simulink model "quadcopter_controly_system"  (R2016b)
settings: Solver=FixedStepAuto  StartTime=0.0  StopTime=30  FixedStep=0.001  MaxStep=0.004  RelTol=1e-3
PreLoadFcn:
  | init
model workspace (MAT data in the model file):
  SL_ROS_VariableLengthArrays_MaxSizes.CommonInfo.ArrayTruncateAction = 'EmitWarning'
  SL_ROS_VariableLengthArrays_MaxSizes.MsgTypeMap = containers.Map
  SL_ROS_VariableLengthArrays_MaxSizes.MsgTypeMap.serialization.keys = {}
  SL_ROS_VariableLengthArrays_MaxSizes.MsgTypeMap.serialization.values = {}
  SL_ROS_VariableLengthArrays_MaxSizes.MsgTypeMap.serialization.uniformity = 0
  SL_ROS_VariableLengthArrays_MaxSizes.MsgTypeMap.serialization.keyType = 'char'
  SL_ROS_VariableLengthArrays_MaxSizes.MsgTypeMap.serialization.valueType = 'any'
undefined symbols (not defined in the file or in its folder): Data, Data_SL_Info
libraries: robotlib x3
settings Model: Creator=ADAM  LastModifiedBy=consti
settings SolverCC: ExtrapolationOrder=1
settings DataIOCC: MaxDataPoints=1  SaveFormat=Structure  SignalLoggingSaveFormat=ModelDataLogs  SaveOutput=off  SignalLogging=off  DSMLogging=off  SaveTime=off  OutputSaveName=model_out  SignalLoggingName=model_out
settings OptimizationCC: ExpressionDepthLimit=2147483647  LifeSpan=inf  SimCompilerOptimization=on
settings DebuggingCC: UnderspecifiedInitializationDetection=Classic  MergeDetectMultiDrivingBlocksExec=none  InheritedTsInSrcMsg=none  MultiTaskDSMMsg=warning  MultiTaskCondExecSysMsg=none  UnconnectedInputMsg=none  UnconnectedOutputMsg=none  UnconnectedLineMsg=none  StateNameClashWarn=warning  SFUnexpectedBacktrackingDiag=warning  SFNoUnconditionalDefaultTransitionDiag=warning  SFExecutionAtInitializationDiag=none
settings HardwareCC: ProdBitPerPointer=32  ProdBitPerSizeT=32  ProdBitPerPtrDiffT=32  ProdLargestAtomicFloat=None  ProdWordSize=32  ProdHWDeviceType=Generic->32-bit x86 compatible
settings ModelReferenceCC: UpdateModelReferenceTargets=IfOutOfDate  PropagateSignalLabelsOutOfModel=off
settings CodeAppCC: MaxIdLength=95
settings GRTTargetCC: TargetLangStandard=C89/C90 (ANSI)  GeneratePreprocessorConditionals=Disable all
settings ConfigComp: CovMetricSettings=dw  CovHtmlReporting=on  CovSaveCumulativeToWorkspaceVar=on  CovSaveSingleToWorkspaceVar=on  CovExternalEMLEnable=off  CovSFcnEnable=off

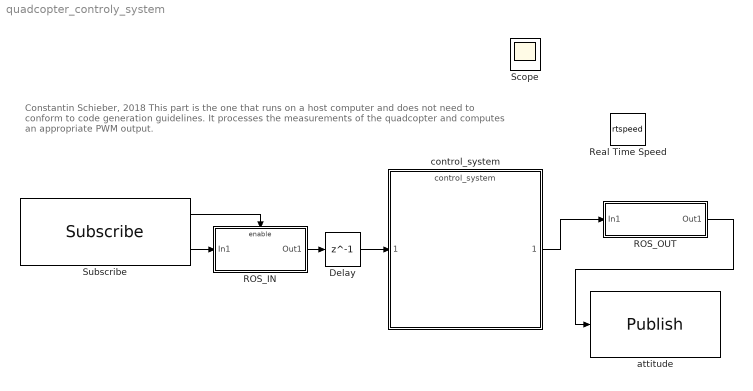
== system quadcopter_controly_system ==
  note: Constantin Schieber, 2018
      |
      | This part is the one that runs on a host computer and does not need to conform to code generation guidelines.
      | It processes the measurements of the quadcopter and computes an appropriate PWM output.
  Delay : Delay  DelayLength=1
  ROS_IN : Subsystem
  ROS_OUT : Subsystem
  Real Time Speed : S-Function  FunctionName=rtspeed  Parameters=speed  SFunctionDeploymentMode=off  EnableBusSupport=off  mask(Simulink Realtime Synchronization){speed=1}
      mask prompts: speed "Simulation Speed (1 = realtime)"
      mask help: Slows down simulation to desired real time speed.
      mask Display:
      | ang=(0:0.0125:1)*2*pi;
      | xp=100*cos(ang);
      | yp=100*sin(ang);
      | plot(-145,-130,155,170,xp,yp,[0 0 70*sqrt(2)/2],[70 0 70*sqrt(2)/2],[-40 40 40 -40 -40],[150 150 120 120 150],[-15 -15],[120 98.5],[15 15],[120 98.5],[100*cos((45+9)/180*pi) 100*cos((45+9)/180*pi)+30 100*cos((45-9)/180*pi)+30 100*cos((45-9)/180*pi)],[100*sin((45+9)/180*pi) 100*sin((45+9)/180*pi)+30 100*sin((45-9)/180*pi)+30 100*sin((45-9)/180*pi)]);
  Subscribe : robotlib/Subscribe  SourceLibraryInfo=This block requires Robotics System Toolbox  topicSource=Specify your own  topic=/dyn_model_measurments  messageType=std_msgs/Float32MultiArray  sampleTime=-1  messageQueueLength=1
  attitude : robotlib/Publish  SourceLibraryInfo=This block requires Robotics System Toolbox  topicSource=Specify your own  topic=/control_system_pwm  messageType=std_msgs/Float32MultiArray  messageQueueLength=1
  control_system : ModelReference  ModelNameDialog=control_system  SimulationMode=Normal  ModelReferenceVersion=1.2838
  Scope : Scope
  wires:
  Delay/1 -> control_system/1
  Subscribe/1 -> ROS_IN/Enable
  Subscribe/2 -> ROS_IN/1(In1)
  ROS_IN/1(Out1) -> Delay/1
  control_system/1 -> ROS_OUT/1(In1)
  ROS_OUT/1(Out1) -> attitude/1

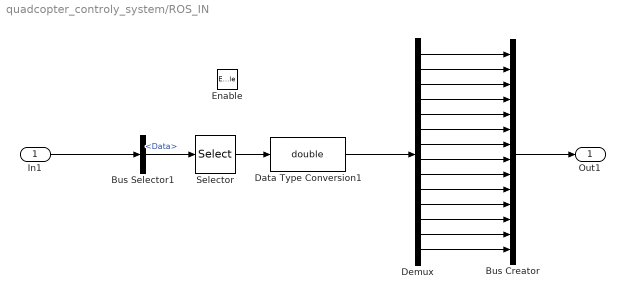
== system quadcopter_controly_system/ROS_IN ==
  In1 : Inport
  Enable : EnablePort
  Bus Creator : BusCreator  Inputs=14
  Bus Selector1 : BusSelector  OutputSignals=Data
  Data Type Conversion1 : DataTypeConversion  OutDataTypeStr=double
  Demux : Demux  Outputs=14
  Selector : Selector  InputPortWidth=128  IndexOptions=Index vector (dialog)  Indices=[1 2 3 4 5 6 7 8 9 10 11 12 13 14]  OutputSizes=1
  Out1 : Outport
  wires:
  Bus Selector1/1 -> Selector/1  "<Data>"
  Demux/10 -> Bus Creator/10
  Demux/3 -> Bus Creator/3
  Demux/9 -> Bus Creator/9
  Selector/1 -> Data Type Conversion1/1
  Data Type Conversion1/1 -> Demux/1
  Demux/4 -> Bus Creator/4
  Demux/8 -> Bus Creator/8
  Demux/6 -> Bus Creator/6
  Demux/14 -> Bus Creator/14
  Demux/7 -> Bus Creator/7
  Demux/13 -> Bus Creator/13
  Bus Creator/1 -> Out1/1
  Demux/11 -> Bus Creator/11
  In1/1 -> Bus Selector1/1
  Demux/2 -> Bus Creator/2
  Demux/12 -> Bus Creator/12
  Demux/5 -> Bus Creator/5
  Demux/1 -> Bus Creator/1

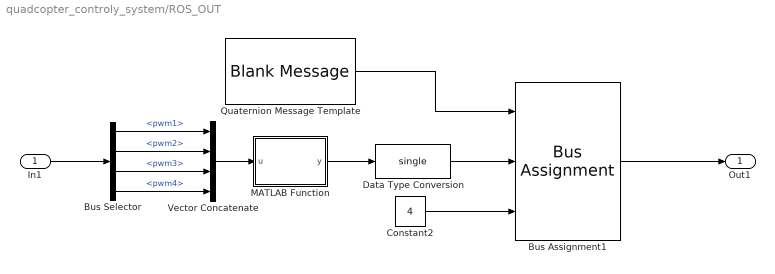
== system quadcopter_controly_system/ROS_OUT ==
  In1 : Inport
  Bus Assignment1 : BusAssignment  AssignedSignals=Data,Data_SL_Info.CurrentLength
  Bus Selector : BusSelector  OutputSignals=pwm1,pwm2,pwm3,pwm4
  Constant2 : Constant  Value=4  OutDataTypeStr=uint32
  Data Type Conversion : DataTypeConversion  OutDataTypeStr=single
  MATLAB Function : MATLAB Function  TreatAsAtomicUnit=on
  Quaternion Message Template : robotlib/Blank Message  SourceLibraryInfo=This block requires Robotics System Toolbox  messageType=std_msgs/Float32MultiArray  SampleTime=inf
  Vector Concatenate : Concatenate  NumInputs=4
  Out1 : Outport
  wires:
  MATLAB Function/1(y) -> Data Type Conversion/1
  Quaternion Message Template/1 -> Bus Assignment1/1
  Data Type Conversion/1 -> Bus Assignment1/2
  In1/1 -> Bus Selector/1
  Bus Selector/1 -> Vector Concatenate/1  "<pwm1>"
  Vector Concatenate/1 -> MATLAB Function/1(u)
  Bus Assignment1/1 -> Out1/1
  Bus Selector/3 -> Vector Concatenate/3  "<pwm3>"
  Bus Selector/4 -> Vector Concatenate/4  "<pwm4>"
  Bus Selector/2 -> Vector Concatenate/2  "<pwm2>"
  Constant2/1 -> Bus Assignment1/3

== matlab function quadcopter_controly_system/ROS_OUT/MATLAB Function ==
  data: u input; y output
function y = fcn(u)


y = zeros(1,128);
for i = 1:4
    y(i) = u(i);
end
end
